simulink model "week2_2"  (R2020b)
settings: Solver=VariableStepAuto  StartTime=0.0  StopTime=10.0  RelTol=1e-3
PreLoadFcn:
  | R=1;
  | be=2;
  | bv=1;
  | Ie=1;
  | Iv=5;
model workspace (MAT data in the model file):
  Fn = Simulink.Parameter
  Fn.Value = [0  0; 1  0.8; 2  1.6; 3  1.6; 4  1.6; 5  1.6; 6  0.8; 7  0; 8  0; 9  0; 10  0]
  Fn.DataType = 'auto'
  Fn.Dimensions = [11 2]
  R = Simulink.Parameter
  R.Value = 1
  R.DataType = 'auto'
  R.Dimensions = [1 1]
  Tin = Simulink.Parameter
  Tin.Value = [1  2; 2  2; 3  2; 4  2; 5  2; 6  0; 7  0; 8  0; 9  0; 10  0]
  Tin.DataType = 'auto'
  Tin.Dimensions = [10 2]
  be = Simulink.Parameter
  be.Value = 2
  be.DataType = 'auto'
  be.Dimensions = [1 1]
  bv = Simulink.Parameter
  bv.Value = 1
  bv.DataType = 'auto'
  bv.Dimensions = [1 1]
  f1 = Simulink.Parameter
  f1.Value = [1; 6; 11; 16; 21; 26; 31; 36; 41; 46; 51]
  f1.DataType = 'auto'
  f1.Dimensions = [11 1]
  le = Simulink.Parameter
  le.Value = 1
  le.DataType = 'auto'
  le.Dimensions = [1 1]
  lv = Simulink.Parameter
  lv.Value = 5
  lv.DataType = 'auto'
  lv.Dimensions = [1 1]
  muk = Simulink.Parameter
  muk.Value = 1
  muk.DataType = 'auto'
  muk.Dimensions = [1 1]
  mus = Simulink.Parameter
  mus.Value = 1.5
  mus.DataType = 'auto'
  mus.Dimensions = [1 1]
settings Model: Creator=hp  LastModifiedBy=hp

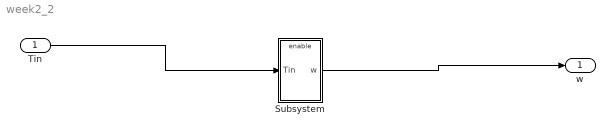
== system week2_2 ==
  Tin : Inport
  Subsystem : Subsystem
  w : Outport
  wires:
  Tin/1 -> Subsystem/1(Tin)
  Subsystem/1(w) -> w/1

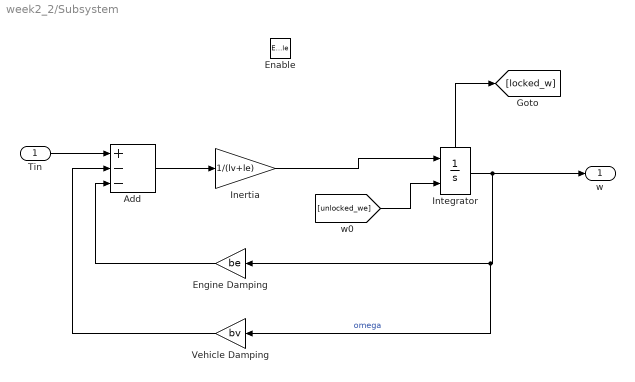
== system week2_2/Subsystem ==
  Tin : Inport
  Enable : EnablePort
  Add : Sum  Inputs=+--
  Engine Damping : Gain  Gain=be
  Inertia : Gain  Gain=1/(lv+le)
  Integrator : Integrator  InitialConditionSource=external  ShowStatePort=on
  Vehicle Damping : Gain  Gain=bv
  w : Outport
  wires:
  Add/1 -> Inertia/1
  Vehicle Damping/1 -> Add/2
  Engine Damping/1 -> Add/3
  Tin/1 -> Add/1
  Integrator/1 -> w/1, Vehicle Damping/1, Engine Damping/1  "omega"
  Integrator/State -> [locked_w]
  [unlocked_we] -> Integrator/2
  Inertia/1 -> Integrator/1
